simulink model "exercise2"  (R2017a)
settings: Solver=VariableStepAuto  StartTime=0.0  StopTime=20  RelTol=1e-3
settings Model: Creator=viktor  LastModifiedBy=viktor

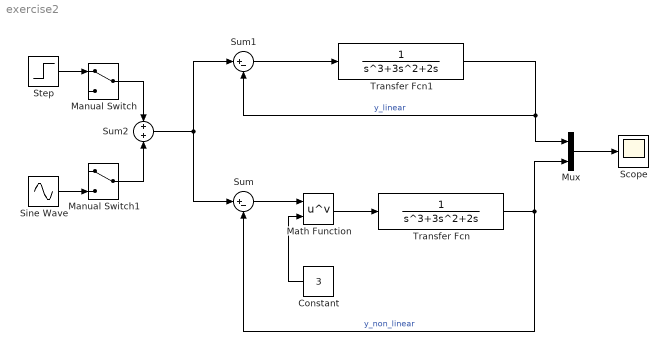
== system exercise2 ==
  Constant : Constant  Value=3
  Manual Switch : ManualSwitch
  Manual Switch1 : ManualSwitch
  Math Function : Math  Operator=pow  SaturateOnIntegerOverflow=on
  Mux : Mux  Inputs=2
  Scope : Scope
  Sine Wave : Sin  Amplitude=0.5  Frequency=10  Phase=2/pi  SampleTime=0
  Step : Step  After=2  SampleTime=0
  Sum : Sum  Inputs=|+-
  Sum1 : Sum  Inputs=|+-
  Sum2 : Sum
  Transfer Fcn : TransferFcn  Denominator=[1 3 2 0]
  Transfer Fcn1 : TransferFcn  Denominator=[1 3 2 0]
  wires:
  Sum/1 -> Math Function/1
  Transfer Fcn/1 -> Sum/2, Mux/2  "y_non_linear"
  Constant/1 -> Math Function/2
  Math Function/1 -> Transfer Fcn/1
  Transfer Fcn1/1 -> Mux/1, Sum1/2  "y_linear"
  Sum1/1 -> Transfer Fcn1/1
  Mux/1 -> Scope/1
  Step/1 -> Manual Switch/1
  Manual Switch/1 -> Sum2/1
  Manual Switch1/1 -> Sum2/2
  Sine Wave/1 -> Manual Switch1/2
  Sum2/1 -> Sum/1, Sum1/1
